simulink model "simulink_problem_1"  (R2022b)
settings: Solver=VariableStepAuto  StartTime=0.0  StopTime=10.0  RelTol=1e-3
settings Model: Creator=Administrator  LastModifiedBy=Administrator

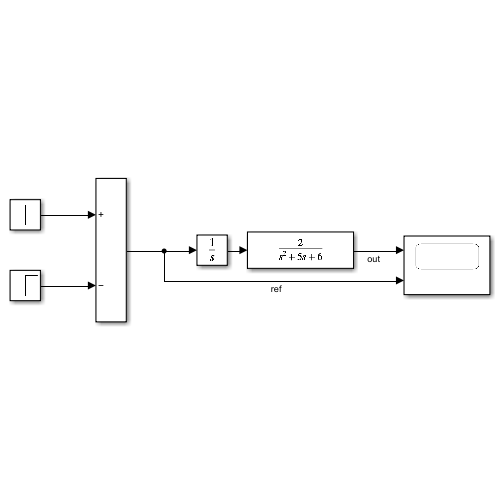
[thumbnail: Simulink's stored preview of the top-level diagram]
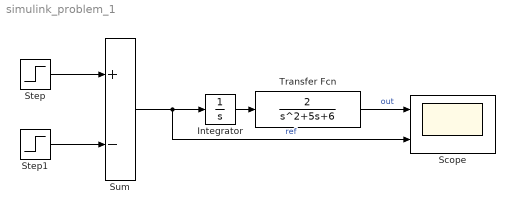
== system simulink_problem_1 ==
  Integrator : Integrator  InitialCondition=4
  Scope : Scope  NumInputPorts=2
  Step : Step  Time=0  SampleTime=0
  Step1 : Step  Time=3  SampleTime=0
  Sum : Sum  Inputs=+-
  Transfer Fcn : TransferFcn  Numerator=[0 0 2]  Denominator=[1 5 6]
  wires:
  Step1/1 -> Sum/2
  Step/1 -> Sum/1
  Sum/1 -> Integrator/1, Scope/2  "ref"
  Transfer Fcn/1 -> Scope/1  "out"
  Integrator/1 -> Transfer Fcn/1
